simulink model "ModelGreenhouseControlSoln"  (R2023b)
settings: Solver=FixedStepAuto  StartTime=0.0  StopTime=inf  RelTol=1e-3
libraries: Arduino_Additional_Lib x1, arduinolib x1
settings Model: ExtModeTrigDuration=2  Creator=nroberts  LastModifiedBy=vboutrou
settings SolverCC: PositivePriorityOrder=on
settings OptimizationCC: EnhancedBackFolding=on  PassReuseOutputArgsAs=Individual arguments  ZeroExternalMemoryAtStartup=off  ZeroInternalMemoryAtStartup=off  MaxStackSize=64  OptimizeBlockOrder=speed  DifferentSizesBufferReuse=on  OptimizationCustomize=off  EfficientTunableParamExpr=on
settings DebuggingCC: ParameterTunabilityLossMsg=error
settings HardwareCC: ProdBitPerInt=16  ProdBitPerPointer=16  ProdBitPerSizeT=16  ProdBitPerPtrDiffT=16  ProdLargestAtomicFloat=None  ProdWordSize=8  ProdHWDeviceType=Atmel->AVR
settings ModelReferenceCC: ModelReferenceNumInstancesAllowed=Single
settings SFSimCC: MATLABDynamicMemAlloc=off
settings RTWCC: Description=Embedded Coder  SystemTargetFile=ert.tlc  HardwareBoard=Arduino Uno  TemplateMakefile=ert_default_tmf  Toolchain=Arduino AVR  BuildConfiguration=Faster Runs
settings CodeAppCC: ForceParamTrailComments=on  IgnoreCustomStorageClasses=off  MaxIdLength=95  OperatorAnnotations=on  SimulinkDataObjDesc=on  SFDataObjDesc=on  InsertBlockDesc=on
settings ERTTargetCC: SupportContinuousTime=on  SupportVariableSizeSignals=on  ExtModeTransport=3  ExtModeStaticAlloc=on  ExtModeAutomaticAllocSize=off  ExtModeStaticAllocSize=250  ExtModeMexFile=ext_xcp  ExtModeIntrfLevel=Level2 - Open

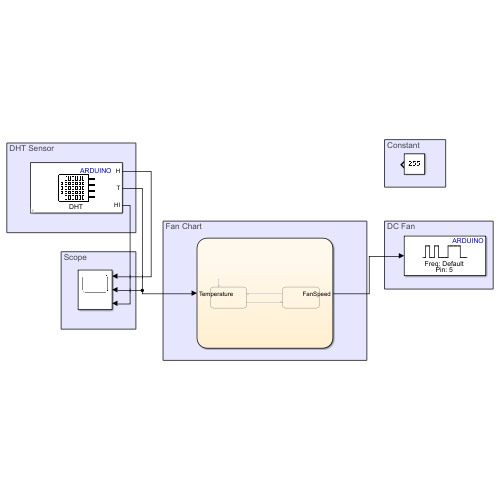
[thumbnail: Simulink's stored preview of the top-level diagram]
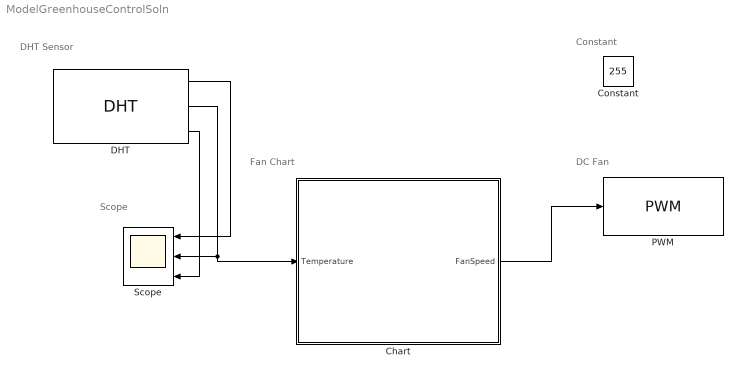
== system ModelGreenhouseControlSoln ==
  note: DC Fan
  note: Constant
  note: Fan Chart
  note: Scope
  note: DHT Sensor
  Chart : Stateflow chart  TreatAsAtomicUnit=on
  Constant : Constant  Value=255
  DHT : Arduino_Additional_Lib/DHT  F=on  Pin=2  Tp=11  Ts=0.5
      settings: SourceProductName=Arduino Additional Sensors Library
  PWM : arduinolib/PWM  pinNumber=5  frequencyType=Default  desiredFrequency=490.2  achievableFrequency=490.2
  Scope : Scope  NumInputPorts=3
  wires:
  DHT/1 -> Scope/1
  DHT/2 -> Chart/1(Temperature), Scope/2
  DHT/3 -> Scope/3
  Chart/1(FanSpeed) -> PWM/1

== stateflow chart ModelGreenhouseControlSoln/Chart ==
  state InitialState
    FanSpeed = 0;
  state ActivatedState
    FanSpeed = 255;
  (default) -> InitialState
  ActivatedState -> InitialState : [Temperature<= 75]
  InitialState -> ActivatedState : [Temperature >= 80]
  data: Temperature input; FanSpeed output
